simulink model "Component"  (R2020a)
settings: Solver=VariableStepAuto  StartTime=0.0  StopTime=10.0  RelTol=1e-3
libraries: fl_lib x1
settings Model: Creator=ivanl  LastModifiedBy=ivanl

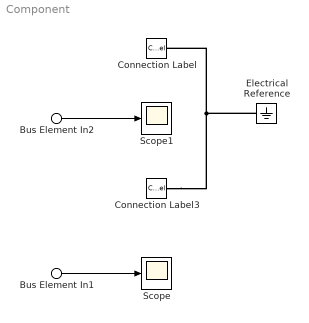
== system Component ==
  Bus Element In2 : Inport  PortName=InBus1
  Bus Element In1 : Inport  Port=2  PortName=InBus
  Connection Label : ConnectionLabel  Label=P1
  Connection Label3 : ConnectionLabel  Label=P2
  Electrical Reference : fl_lib/Electrical/Electrical Elements/Electrical Reference
  Scope : Scope
  Scope1 : Scope
  wires:
  Bus Element In1/1 -> Scope/1
  Bus Element In2/1 -> Scope1/1
  connections:
  Electrical Reference/LConn1 -- Connection Label/LConn1 -- Connection Label3/LConn1
